simulink model "ABS_SISO_SlipStateIOFBLModel_gamma"  (Simulink 7.1)
settings: Solver=ode45  StartTime=0.0  StopTime=3.4  RelTol=1e-3
values from neighbouring files (symbols this model uses):
  Bf = 0.08    [ABS_set_param.m]
  Cs = 1050.0    (= 1050)    [ABS_set_param.m]    (also in gamma_driven_suspension.m)
  Ct = 1500.0    (= 1500)    [ABS_set_param.m]
  Cx = 0.856    [ABS_set_param.m]
  Fz = Mt*g    (= 4316.4)    [ABS_set_param.m]
  Im = I    (= 1.6)    [ABS_set_param.m]
  Ks = 19960.0    (= 19960)    [ABS_set_param.m]    (also in gamma_driven_suspension.m)
  Kw = 175500.0    (= 175500)    [ABS_set_param.m]    (also in gamma_driven_suspension.m)
  l_0 = 0.20    (= 0.2)    [ABS_set_param.m]
  ms = 427.0    (= 427)    [ABS_set_param.m]    (also in gamma_driven_suspension.m)
  Mt = M    (= 440)    [ABS_set_param.m]
  mu_0 = 0.9    [ABS_set_param.m]
  mw = 40.0    (= 40)    [ABS_set_param.m]    (also in gamma_driven_suspension.m)
  R0 = 0.35    [ABS_set_param.m]
  v_initial = 120000/(3600)    (= 33.3333333333)    [ABS_set_param.m]
  w_initial = v_initial/R0    (= 95.2380952381)    [ABS_set_param.m]
settings Model: Creator=Nyandoro  LastModifiedBy=theShunainai
settings OptimizationCC: InitFltsAndDblsToZero=off

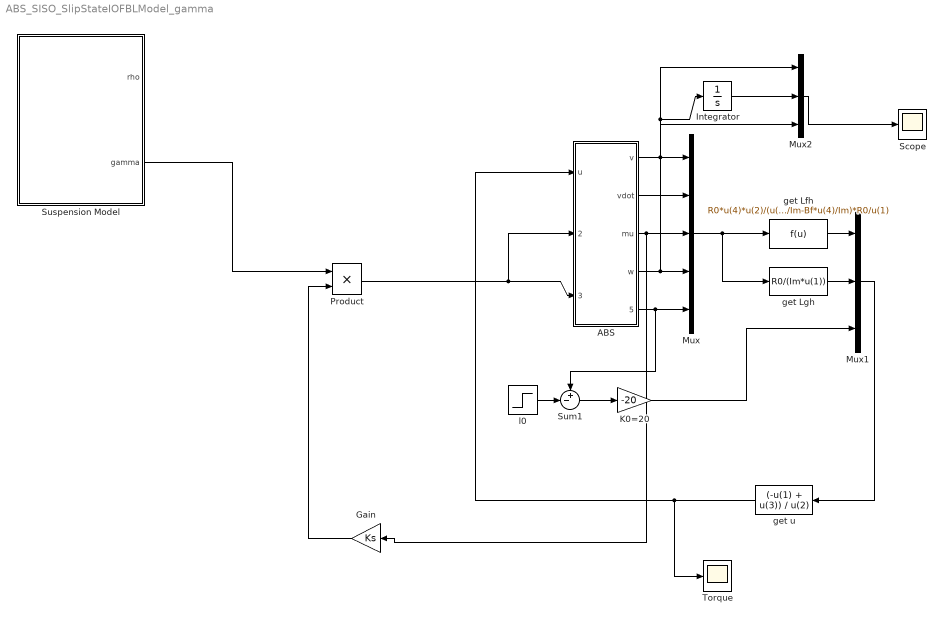
== system ABS_SISO_SlipStateIOFBLModel_gamma ==
  ABS : Subsystem
  Gain : Gain  Orientation=left  Gain=Ks  ParameterDataType=sfix(16)  ParameterScaling=2^0  OutDataType=sfix(16)  OutScaling=2^0
  Integrator : Integrator
  K0=20 : Gain  Gain=-20  ParameterDataType=sfix(16)  ParameterScaling=2^0  OutDataType=sfix(16)  OutScaling=2^0
  Mux : Mux  Inputs=5
  Mux1 : Mux  Inputs=3
  Mux2 : Mux  Inputs=3
  Product : Product  OutDataType=sfix(16)  OutScaling=2^0  RndMeth=Zero
  Scope : Scope
      settings: SaveName=ScopeData4
  Sum1 : Sum  Inputs=+-|  OutDataType=sfix(16)  OutScaling=2^0
  Suspension Model : Subsystem
  Torque : Scope
      settings: SaveName=ScopeData2
  get Lfh : Fcn  Expr=R0*u(4)*u(2)/(u(1)^2) - (u(3)*Fz*R0/Im-Bf*u(4)/Im)*R0/u(1)
  get Lgh : Fcn  Expr=R0/(Im*u(1))
  get u : Fcn  Orientation=left  Expr=(-u(1) + u(3)) / u(2)
  l0 : Step  Time=0  After=l_0  SampleTime=0
  wires:
  ABS/1(v) -> Mux/1, Mux2/1, Integrator/1
  ABS/2(vdot) -> Mux/2
  ABS/3(mu) -> Mux/3, Gain/1
  ABS/4(w) -> Mux/4, Mux2/3
  Mux/1 -> get Lfh/1, get Lgh/1
  ABS/5(lambda) -> Mux/5, Sum1/1
  l0/1 -> Sum1/2
  Sum1/1 -> K0=20/1
  get Lfh/1 -> Mux1/1
  get Lgh/1 -> Mux1/2
  K0=20/1 -> Mux1/3
  Mux1/1 -> get u/1
  get u/1 -> ABS/1(u), Torque/1
  Integrator/1 -> Mux2/2
  Mux2/1 -> Scope/1
  Gain/1 -> Product/2
  Suspension Model/2(gamma) -> Product/1
  Product/1 -> ABS/3(gamma2), ABS/2(gamma 1)

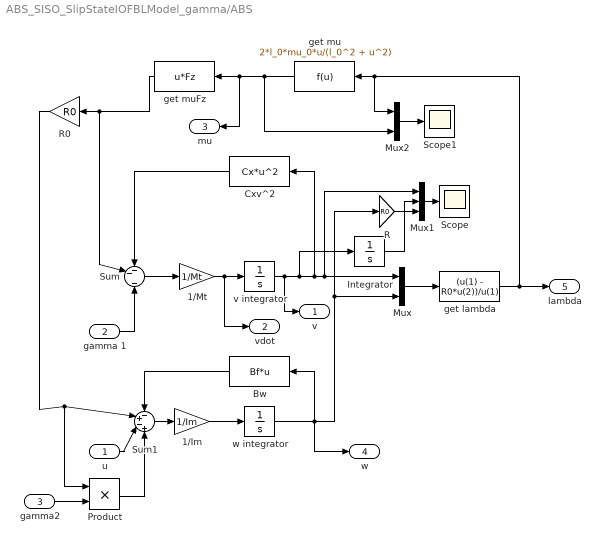
== system ABS_SISO_SlipStateIOFBLModel_gamma/ABS ==
  u : Inport
  gamma 1 : Inport  Port=2  OutDataType=sfix(16)  OutScaling=2^0
  gamma2 : Inport  Port=3  OutDataType=sfix(16)  OutScaling=2^0
  1/Im : Gain  Gain=1/Im  ParameterDataType=sfix(16)  ParameterScaling=2^0  OutDataType=sfix(16)  OutScaling=2^0
  1/Mt : Gain  Gain=1/Mt  ParameterDataType=sfix(16)  ParameterScaling=2^0  OutDataType=sfix(16)  OutScaling=2^0
  Bw : Fcn  Orientation=left  Expr=Bf*u
  Cxv^2 : Fcn  Orientation=left  Expr=Cx*u^2
  Integrator : Integrator
  Mux : Mux  Inputs=2
  Mux1 : Mux  Inputs=3
  Mux2 : Mux  Inputs=2
  Product : Product  OutDataType=sfix(16)  OutScaling=2^0  RndMeth=Zero
  R : Gain  Gain=R0  ParameterDataType=sfix(16)  ParameterScaling=2^0  OutDataType=sfix(16)  OutScaling=2^0
  R0 : Gain  Orientation=left  Gain=R0  ParameterDataType=sfix(16)  ParameterScaling=2^0  OutDataType=sfix(16)  OutScaling=2^0
  Scope : Scope
  Scope1 : Scope
  Sum : Sum  Inputs=--|-  OutDataType=sfix(16)  OutScaling=2^0
  Sum1 : Sum  Inputs=-+-+  OutDataType=sfix(16)  OutScaling=2^0
  get lambda : Fcn  Expr=(u(1) - R0*u(2))/u(1)
  get mu : Fcn  Orientation=left  Expr=2*l_0*mu_0*u/(l_0^2 + u^2)
  get muFz : Fcn  Orientation=left  Expr=u*Fz
  v integrator : Integrator  InitialCondition=v_initial
  w integrator : Integrator  InitialCondition=w_initial  LimitOutput=on  LowerSaturationLimit=0
  v : Outport  OutDataType=sfix(16)  OutScaling=2^0
  vdot : Outport  Port=2  OutDataType=sfix(16)  OutScaling=2^0
  mu : Outport  Orientation=left  Port=3  OutDataType=sfix(16)  OutScaling=2^0
  w : Outport  Port=4  OutDataType=sfix(16)  OutScaling=2^0
  lambda : Outport  Port=5  OutDataType=sfix(16)  OutScaling=2^0
  wires:
  v integrator/1 -> v/1, Cxv^2/1, Mux/1, Mux1/1, Integrator/1
  Cxv^2/1 -> Sum/1
  1/Mt/1 -> v integrator/1, vdot/1
  Sum/1 -> 1/Mt/1
  w integrator/1 -> Bw/1, Mux/2, R/1, w/1
  Mux/1 -> get lambda/1
  get lambda/1 -> get mu/1, Mux2/1, lambda/1
  get mu/1 -> Mux2/2, mu/1, get muFz/1
  Sum1/1 -> 1/Im/1
  Bw/1 -> Sum1/1
  R0/1 -> Sum1/2, Product/1
  1/Im/1 -> w integrator/1
  Mux1/1 -> Scope/1
  R/1 -> Mux1/2
  Mux2/1 -> Scope1/1
  u/1 -> Sum1/3
  get muFz/1 -> R0/1, Sum/2
  Integrator/1 -> Mux1/3
  gamma 1/1 -> Sum/3
  gamma2/1 -> Product/2
  Product/1 -> Sum1/4

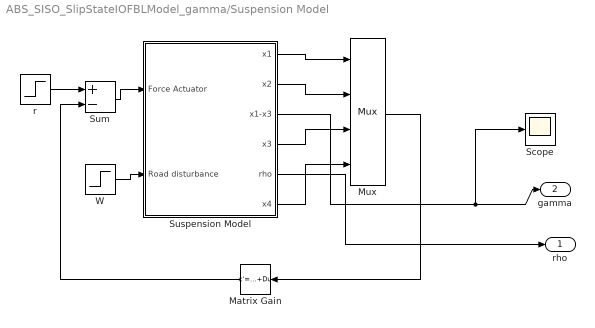
== system ABS_SISO_SlipStateIOFBLModel_gamma/Suspension Model ==
  Matrix Gain : StateSpace  Orientation=left  A=[]  B=[]  C=[]  D=K  mask(Matrix Gain){@1=-Kgamma}
      mask prompts: @1 "Gain matrix:"
      mask help: Matrix Gain.
      mask init:
      | K=@1;
      mask Help: Multiplies input vector by entered matrix to produce output vector (y=Au).
      mask Display: disp('K')
  Mux : Mux
  Scope : Scope
      settings: YMin=0.0175  YMax=0.0425  SaveName=ScopeData3
  Sum : Sum  Inputs=+-  SaturateOnIntegerOverflow=on  InputSameDT=on  OutDataTypeStr=Inherit: Same as first input
  Suspension Model : Subsystem
  W : Step  Time=0  After=-.1
  r : Step  Time=0  After=0
  rho : Outport  OutDataType=sfix(16)  OutScaling=2^0
  gamma : Outport  Port=2  OutDataType=sfix(16)  OutScaling=2^0
  wires:
  W/1 -> Suspension Model/2(Road disturbance)
  Sum/1 -> Suspension Model/1(Force Actuator)
  r/1 -> Sum/1
  Matrix Gain/1 -> Sum/2
  Mux/1 -> Matrix Gain/1
  Suspension Model/1(x1) -> Mux/1
  Suspension Model/2(x2) -> Mux/2
  Suspension Model/4(x3) -> Mux/3
  Suspension Model/6(x4) -> Mux/4
  Suspension Model/3(x1-x3) -> gamma/1, Scope/1
  Suspension Model/5(rho) -> rho/1

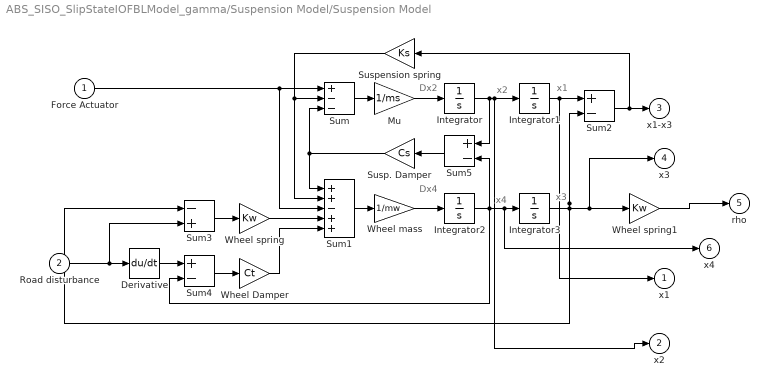
== system ABS_SISO_SlipStateIOFBLModel_gamma/Suspension Model/Suspension Model ==
  note: x3
  note: x4
  note: Dx4
  note: x1
  note: x2
  note: Dx2
  Force Actuator : Inport
  Road disturbance : Inport  Port=2
  Derivative : Derivative
  Integrator{,1..3} (4 alike) : Integrator
  Mu : Gain  Gain=1/ms  SaturateOnIntegerOverflow=on  OutDataTypeStr=Inherit: Same as input  ParamDataTypeStr=Inherit: Same as input
  Sum : Sum  Inputs=+--  SaturateOnIntegerOverflow=on  InputSameDT=on  OutDataTypeStr=Inherit: Same as first input
  Sum1 : Sum  Inputs=++-++  SaturateOnIntegerOverflow=on  InputSameDT=on  OutDataTypeStr=Inherit: Same as first input
  Sum2 : Sum  Inputs=+-  SaturateOnIntegerOverflow=on  InputSameDT=on  OutDataTypeStr=Inherit: Same as first input
  Sum3 : Sum  Inputs=-+  SaturateOnIntegerOverflow=on  InputSameDT=on  OutDataTypeStr=Inherit: Same as first input
  Sum4 : Sum  Inputs=+-  SaturateOnIntegerOverflow=on  InputSameDT=on  OutDataTypeStr=Inherit: Same as first input
  Sum5 : Sum  Orientation=left  Inputs=+-  SaturateOnIntegerOverflow=on  InputSameDT=on  OutDataTypeStr=Inherit: Same as first input
  Susp. Damper : Gain  Orientation=left  Gain=Cs  SaturateOnIntegerOverflow=on  OutDataTypeStr=Inherit: Same as input  ParamDataTypeStr=Inherit: Same as input
  Suspension spring : Gain  Orientation=left  Gain=Ks  SaturateOnIntegerOverflow=on  OutDataTypeStr=Inherit: Same as input  ParamDataTypeStr=Inherit: Same as input
  Wheel Damper : Gain  Gain=Ct  SaturateOnIntegerOverflow=on  OutDataTypeStr=Inherit: Same as input  ParamDataTypeStr=Inherit: Same as input
  Wheel mass : Gain  Gain=1/mw  SaturateOnIntegerOverflow=on  OutDataTypeStr=Inherit: Same as input  ParamDataTypeStr=Inherit: Same as input
  Wheel spring : Gain  Gain=Kw  SaturateOnIntegerOverflow=on  OutDataTypeStr=Inherit: Same as input  ParamDataTypeStr=Inherit: Same as input
  Wheel spring1 : Gain  Gain=Kw  SaturateOnIntegerOverflow=on  OutDataTypeStr=Inherit: Same as input  ParamDataTypeStr=Inherit: Same as input
  x1 : Outport  InitialOutput=0
  x2 : Outport  Port=2  InitialOutput=0
  x1-x3 : Outport  Port=3  InitialOutput=0
  x3 : Outport  Port=4  InitialOutput=0
  rho : Outport  Port=5  InitialOutput=0
  x4 : Outport  Port=6  InitialOutput=0
  wires:
  Integrator3/1 -> Sum3/1, Sum2/2, Wheel spring1/1, x3/1
  Integrator1/1 -> Sum2/1, x1/1
  Sum5/1 -> Susp. Damper/1
  Road disturbance/1 -> Derivative/1, Sum3/2
  Derivative/1 -> Sum4/1
  Force Actuator/1 -> Sum1/3, Sum/1
  Sum4/1 -> Wheel Damper/1
  Sum3/1 -> Wheel spring/1
  Wheel spring/1 -> Sum1/4
  Wheel Damper/1 -> Sum1/5
  Suspension spring/1 -> Sum1/2, Sum/2
  Sum2/1 -> x1-x3/1, Suspension spring/1
  Integrator/1 -> x2/1, Integrator1/1, Sum5/1
  Sum/1 -> Mu/1
  Mu/1 -> Integrator/1
  Susp. Damper/1 -> Sum/3, Sum1/1
  Integrator2/1 -> Sum5/2, Sum4/2, Integrator3/1, x4/1
  Sum1/1 -> Wheel mass/1
  Wheel mass/1 -> Integrator2/1
  Wheel spring1/1 -> rho/1
